simulink model "simulink_model"  (R2018b)
settings: Solver=VariableStepAuto  StartTime=0.0  StopTime=15  RelTol=1e-3
values from neighbouring files (symbols this model uses):
  B = 500    [ode_function.m]    (also in parameters.m; state_space.m = [0 ; 0 ; 0 ; (k2/m2)])
  k1 = 500    [ode_function.m]    (also in parameters.m; state_space.m)
  k2 = 1000    [ode_function.m]    (also in parameters.m; state_space.m)
  m1 = 250    [ode_function.m]    (also in parameters.m; state_space.m)
  m2 = 50    [ode_function.m]    (also in parameters.m; state_space.m)
settings Model: Creator=PC  LastModifiedBy=PC

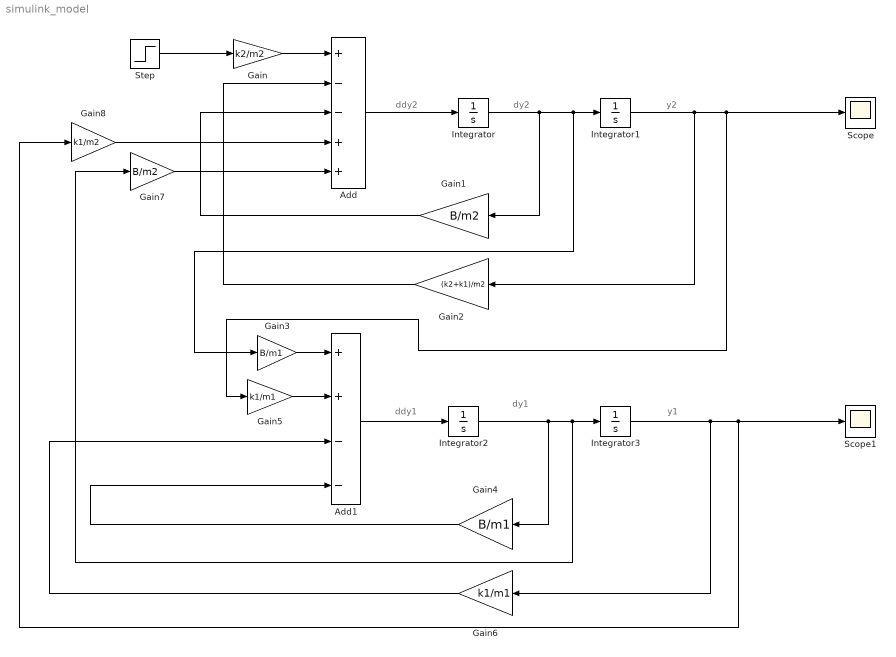
== system simulink_model ==
  note: y1
  note: dy1
  note: ddy1
  note: ddy2
  note: dy2
  note: y2
  Add : Sum  Inputs=+--++
  Add1 : Sum  Inputs=++--
  Gain : Gain  Gain=k2/m2
  Gain1 : Gain  Gain=B/m2
  Gain2 : Gain  Gain=(k2+k1)/m2
  Gain3 : Gain  Gain=B/m1
  Gain4 : Gain  Gain=B/m1
  Gain5 : Gain  Gain=k1/m1
  Gain6 : Gain  Gain=k1/m1
  Gain7 : Gain  Gain=B/m2
  Gain8 : Gain  Gain=k1/m2
  Integrator{,1..3} (4 alike) : Integrator
  Scope : Scope
  Scope1 : Scope
  Step : Step  Time=0  SampleTime=0
  wires:
  Gain/1 -> Add/1
  Add/1 -> Integrator/1
  Gain2/1 -> Add/2
  Gain1/1 -> Add/3
  Add1/1 -> Integrator2/1
  Gain3/1 -> Add1/1
  Gain5/1 -> Add1/2
  Gain4/1 -> Add1/4
  Gain6/1 -> Add1/3
  Gain7/1 -> Add/5
  Gain8/1 -> Add/4
  Step/1 -> Gain/1
  Integrator1/1 -> Gain5/1, Scope/1, Gain2/1
  Integrator2/1 -> Gain4/1, Gain7/1, Integrator3/1
  Integrator3/1 -> Gain8/1, Scope1/1, Gain6/1
  Integrator/1 -> Gain1/1, Gain3/1, Integrator1/1
